simulink model "Gesamtsystem_VirtuelleTestUmgebung"  (R2018b)
settings: Solver=FixedStepDiscrete  StartTime=0.0  StopTime=120  RelTol=1e-3  EnableMultiTasking=on
undefined symbols (not defined in the file): sigbuilder_block
libraries: simulink x2
settings Model: ExtModeTrigDuration=8  Creator=Nici  LastModifiedBy=Nici
settings SolverCC: AutoInsertRateTranBlk=on
settings OptimizationCC: DefaultUnderspecifiedDataType=single  EnhancedBackFolding=on  PassReuseOutputArgsAs=Individual arguments  MaxStackSize=512  OptimizeBlockOrder=speed  DifferentSizesBufferReuse=on  OptimizationCustomize=off
settings DebuggingCC: ParameterTunabilityLossMsg=error  UnderSpecifiedDataTypeMsg=warning
settings HardwareCC: ProdBitPerChar=16  ProdBitPerInt=16  ProdBitPerPointer=32  ProdBitPerSizeT=32  ProdBitPerPtrDiffT=32  ProdLargestAtomicInteger=Integer  ProdLargestAtomicFloat=None  ProdWordSize=16  ProdLongLongMode=on  ProdHWDeviceType=Texas Instruments->C2000
settings SFSimCC: MATLABDynamicMemAlloc=off
settings RTWCC: SystemTargetFile=ert.tlc  HardwareBoard=TI Delfino F2833x  TemplateMakefile=ert_default_tmf  GenerateReport=on  Toolchain=Texas Instruments Code Composer Studio (C2000)  IncludeHyperlinkInReport=on  LaunchReport=on  GenerateTraceInfo=on  GenerateTraceReport=on  GenerateTraceReportSl=on  GenerateTraceReportSf=on  GenerateTraceReportEml=on
settings CodeAppCC: ForceParamTrailComments=on  IgnoreCustomStorageClasses=off  OperatorAnnotations=on  SimulinkDataObjDesc=on  SFDataObjDesc=on  InsertBlockDesc=on
settings ERTTargetCC: CodeReplacementLibrary=TI C28x  SupportContinuousTime=on

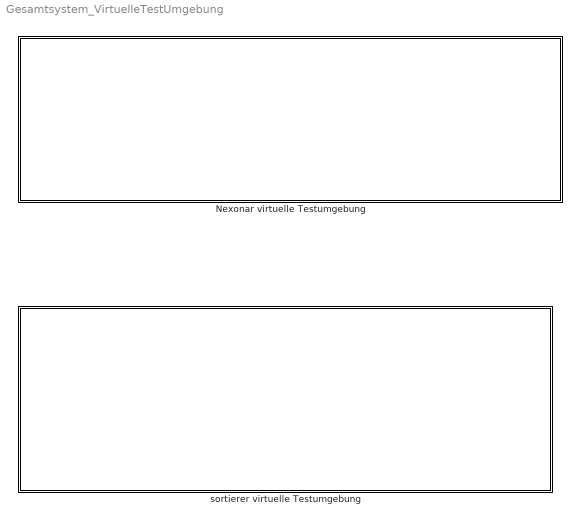
== system Gesamtsystem_VirtuelleTestUmgebung ==
  Nexonar virtuelle Testumgebung : Subsystem
  sortierer virtuelle Testumgebung : Subsystem

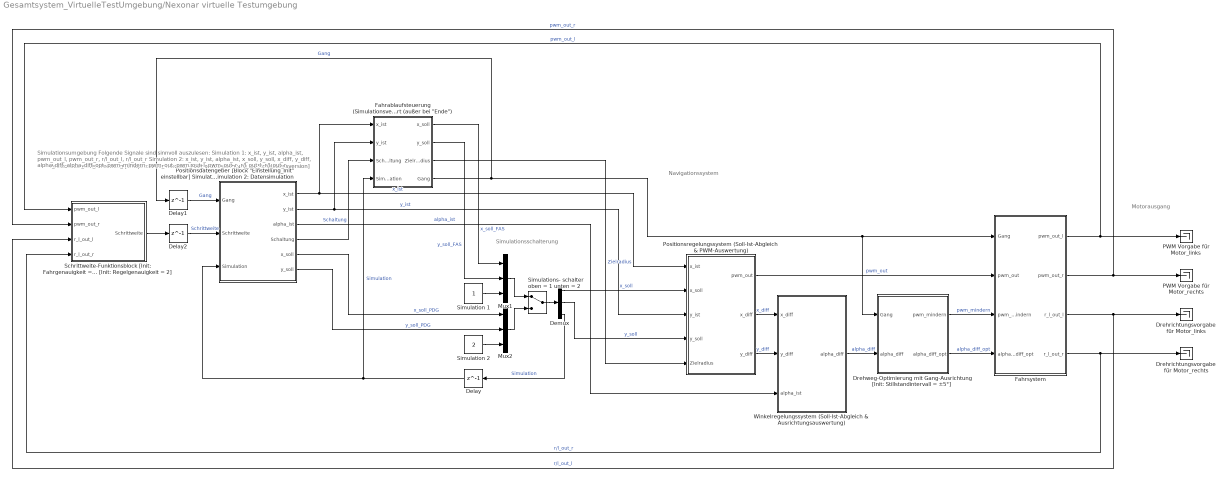
== system Gesamtsystem_VirtuelleTestUmgebung/Nexonar virtuelle Testumgebung ==
  note: Motorausgang
  note: Positionsdatenverarbeitung
      |
      |
      |
      |
      |
      |
      |
      |
      |
      |
      |
      |
      |
      |
      | [entspricht der Nexonar-Positionsbestimmung
      | als Simulationsversion]
  note: Simulationsschalterung
  note: Simulationsumgebung
      |
      |
      |
      |
      |
      |
      |
      |
      |
      |
      |
      |
      |
      |
      |
      |
      |
      |
      |
      |
      |
      |
      |
      |
      |
      |
      |
      |
      |
      |
      | Folgende Signale sind sinnvoll auszulesen:
      | Simulation 1: x_ist, y_ist, alpha_ist, pwm_out_l, pwm_out_r, r/l_out_l, r/l_out_r
      | Simulation 2: x_ist, y_ist, alpha_ist, x_soll, y_soll, x_diff, y_diff, alpha_diff, alpha_diff_opt, pwm_mindern, pwm_out, pwm_out_l, pwm_out_r, r/l_out_l, r/l_out_r
  note: Navigationssystem
  Delay : Delay  DelayLength=1  InitialCondition=0
  Delay1 : Delay  DelayLength=1  InitialCondition=0
  Delay2 : Delay  DelayLength=1  InitialCondition=0
  Demux : Demux  Outputs=3
  Drehrichtungsvorgabe für Motor_links : Terminator
  Drehrichtungsvorgabe für Motor_rechts : Terminator
  Drehweg-Optimierung mit Gang-Ausrichtung [Init: Stillstandintervall = ±5°] : Stateflow chart  TreatAsAtomicUnit=on
  "Fahrablaufsteuerung (Simulationsversion) [Init: Zielradius = 5mm] Gang = 0: vorwaerts Gang = 1: rueckwaerts Folgende Werte fuer den Ablauf sind einstellbar: - Zielkoordinatenwerte - Gangwert (außer bei \"Ende\")" : Stateflow chart  TreatAsAtomicUnit=on
  Fahrsystem : Stateflow chart  TreatAsAtomicUnit=on
  Mux1 : Mux  Inputs=3
  Mux2 : Mux  Inputs=3
  PWM Vorgabe für Motor_links : Terminator
  PWM Vorgabe für Motor_rechts : Terminator
  "Positionsdatengeber [Block \"Einstellung_Init\" einstellbar] Simulation 1: Fahrsimulation Simulation 2: Datensimulation" : Stateflow chart  TreatAsAtomicUnit=on
  Positionsregelungssystem (Soll-Ist-Abgleich & PWM-Auswertung) : Subsystem
  Schrittweite-Funktionsblock [Init: Fahrgenauigkeit = 10] [Init: Drehgenauigkeit = 30] [Init: Regelgenauigkeit = 2] : MATLAB Function  TreatAsAtomicUnit=on
  Simulation 1 : Constant
  Simulation 2 : Constant  Value=2
  Simulations- schalter oben = 1 unten = 2 : ManualSwitch
  Winkelregelungssystem (Soll-Ist-Abgleich & Ausrichtungsauswertung) : Subsystem
  wires:
  "Positionsdatengeber [Block \"Einstellung_Init\" einstellbar] Simulation 1: Fahrsimulation Simulation 2: Datensimulation"/1(x_ist) -> "Fahrablaufsteuerung (Simulationsversion) [Init: Zielradius = 5mm] Gang = 0: vorwaerts Gang = 1: rueckwaerts Folgende Werte fuer den Ablauf sind einstellbar: - Zielkoordinatenwerte - Gangwert (außer bei \"Ende\")"/1(x_ist), Positionsregelungssystem (Soll-Ist-Abgleich & PWM-Auswertung)/1(x_ist)  "x_ist"
  "Positionsdatengeber [Block \"Einstellung_Init\" einstellbar] Simulation 1: Fahrsimulation Simulation 2: Datensimulation"/2(y_ist) -> "Fahrablaufsteuerung (Simulationsversion) [Init: Zielradius = 5mm] Gang = 0: vorwaerts Gang = 1: rueckwaerts Folgende Werte fuer den Ablauf sind einstellbar: - Zielkoordinatenwerte - Gangwert (außer bei \"Ende\")"/2(y_ist), Positionsregelungssystem (Soll-Ist-Abgleich & PWM-Auswertung)/3(y_ist)  "y_ist"
  "Fahrablaufsteuerung (Simulationsversion) [Init: Zielradius = 5mm] Gang = 0: vorwaerts Gang = 1: rueckwaerts Folgende Werte fuer den Ablauf sind einstellbar: - Zielkoordinatenwerte - Gangwert (außer bei \"Ende\")"/2(y_soll) -> Mux1/2  "y_soll_FAS"
  Simulation 1/1 -> Mux1/3
  Positionsregelungssystem (Soll-Ist-Abgleich & PWM-Auswertung)/1(pwm_out) -> Fahrsystem/2(pwm_out)  "pwm_out"
  "Positionsdatengeber [Block \"Einstellung_Init\" einstellbar] Simulation 1: Fahrsimulation Simulation 2: Datensimulation"/4(Schaltung) -> "Fahrablaufsteuerung (Simulationsversion) [Init: Zielradius = 5mm] Gang = 0: vorwaerts Gang = 1: rueckwaerts Folgende Werte fuer den Ablauf sind einstellbar: - Zielkoordinatenwerte - Gangwert (außer bei \"Ende\")"/3(Schaltung)  "Schaltung"
  Delay2/1 -> "Positionsdatengeber [Block \"Einstellung_Init\" einstellbar] Simulation 1: Fahrsimulation Simulation 2: Datensimulation"/2(Schrittweite)  "Schrittweite"
  Delay1/1 -> "Positionsdatengeber [Block \"Einstellung_Init\" einstellbar] Simulation 1: Fahrsimulation Simulation 2: Datensimulation"/1(Gang)  "Gang"
  "Positionsdatengeber [Block \"Einstellung_Init\" einstellbar] Simulation 1: Fahrsimulation Simulation 2: Datensimulation"/3(alpha_ist) -> Winkelregelungssystem (Soll-Ist-Abgleich & Ausrichtungsauswertung)/3(alpha_ist)  "alpha_ist"
  "Positionsdatengeber [Block \"Einstellung_Init\" einstellbar] Simulation 1: Fahrsimulation Simulation 2: Datensimulation"/5(x_soll) -> Mux2/1  "x_soll_PDG"
  Delay/1 -> "Positionsdatengeber [Block \"Einstellung_Init\" einstellbar] Simulation 1: Fahrsimulation Simulation 2: Datensimulation"/3(Simulation), "Fahrablaufsteuerung (Simulationsversion) [Init: Zielradius = 5mm] Gang = 0: vorwaerts Gang = 1: rueckwaerts Folgende Werte fuer den Ablauf sind einstellbar: - Zielkoordinatenwerte - Gangwert (außer bei \"Ende\")"/4(Simulation)  "Simulation"
  "Positionsdatengeber [Block \"Einstellung_Init\" einstellbar] Simulation 1: Fahrsimulation Simulation 2: Datensimulation"/6(y_soll) -> Mux2/2  "y_soll_PDG"
  Drehweg-Optimierung mit Gang-Ausrichtung [Init: Stillstandintervall = ±5°]/2(alpha_diff_opt) -> Fahrsystem/4(alpha_diff_opt)  "alpha_diff_opt"
  Winkelregelungssystem (Soll-Ist-Abgleich & Ausrichtungsauswertung)/1(alpha_diff) -> Drehweg-Optimierung mit Gang-Ausrichtung [Init: Stillstandintervall = ±5°]/2(alpha_diff)  "alpha_diff"
  Fahrsystem/4(r_l_out_r) -> Schrittweite-Funktionsblock [Init: Fahrgenauigkeit = 10] [Init: Drehgenauigkeit = 30] [Init: Regelgenauigkeit = 2]/4(r_l_out_r), Drehrichtungsvorgabe für Motor_rechts/1  "r/l_out_r"
  Mux1/1 -> Simulations- schalter oben = 1 unten = 2/1
  Demux/2 -> Positionsregelungssystem (Soll-Ist-Abgleich & PWM-Auswertung)/4(y_soll)  "y_soll"
  Positionsregelungssystem (Soll-Ist-Abgleich & PWM-Auswertung)/2(x_diff) -> Winkelregelungssystem (Soll-Ist-Abgleich & Ausrichtungsauswertung)/1(x_diff)  "x_diff"
  Fahrsystem/3(r_l_out_l) -> Drehrichtungsvorgabe für Motor_links/1, Schrittweite-Funktionsblock [Init: Fahrgenauigkeit = 10] [Init: Drehgenauigkeit = 30] [Init: Regelgenauigkeit = 2]/3(r_l_out_l)  "r/l_out_l"
  Simulations- schalter oben = 1 unten = 2/1 -> Demux/1
  "Fahrablaufsteuerung (Simulationsversion) [Init: Zielradius = 5mm] Gang = 0: vorwaerts Gang = 1: rueckwaerts Folgende Werte fuer den Ablauf sind einstellbar: - Zielkoordinatenwerte - Gangwert (außer bei \"Ende\")"/4(Gang) -> Drehweg-Optimierung mit Gang-Ausrichtung [Init: Stillstandintervall = ±5°]/1(Gang), Fahrsystem/1(Gang), Delay1/1  "Gang"
  "Fahrablaufsteuerung (Simulationsversion) [Init: Zielradius = 5mm] Gang = 0: vorwaerts Gang = 1: rueckwaerts Folgende Werte fuer den Ablauf sind einstellbar: - Zielkoordinatenwerte - Gangwert (außer bei \"Ende\")"/3(Zielradius) -> Positionsregelungssystem (Soll-Ist-Abgleich & PWM-Auswertung)/5(Zielradius)  "Zielradius"
  Fahrsystem/1(pwm_out_l) -> PWM Vorgabe für Motor_links/1, Schrittweite-Funktionsblock [Init: Fahrgenauigkeit = 10] [Init: Drehgenauigkeit = 30] [Init: Regelgenauigkeit = 2]/1(pwm_out_l)  "pwm_out_l"
  Simulation 2/1 -> Mux2/3
  "Fahrablaufsteuerung (Simulationsversion) [Init: Zielradius = 5mm] Gang = 0: vorwaerts Gang = 1: rueckwaerts Folgende Werte fuer den Ablauf sind einstellbar: - Zielkoordinatenwerte - Gangwert (außer bei \"Ende\")"/1(x_soll) -> Mux1/1  "x_soll_FAS"
  Schrittweite-Funktionsblock [Init: Fahrgenauigkeit = 10] [Init: Drehgenauigkeit = 30] [Init: Regelgenauigkeit = 2]/1(Schrittweite) -> Delay2/1
  Positionsregelungssystem (Soll-Ist-Abgleich & PWM-Auswertung)/3(y_diff) -> Winkelregelungssystem (Soll-Ist-Abgleich & Ausrichtungsauswertung)/2(y_diff)  "y_diff"
  Demux/1 -> Positionsregelungssystem (Soll-Ist-Abgleich & PWM-Auswertung)/2(x_soll)  "x_soll"
  Demux/3 -> Delay/1  "Simulation"
  Drehweg-Optimierung mit Gang-Ausrichtung [Init: Stillstandintervall = ±5°]/1(pwm_mindern) -> Fahrsystem/3(pwm_mindern)  "pwm_mindern"
  Fahrsystem/2(pwm_out_r) -> PWM Vorgabe für Motor_rechts/1, Schrittweite-Funktionsblock [Init: Fahrgenauigkeit = 10] [Init: Drehgenauigkeit = 30] [Init: Regelgenauigkeit = 2]/2(pwm_out_r)  "pwm_out_r"
  Mux2/1 -> Simulations- schalter oben = 1 unten = 2/2

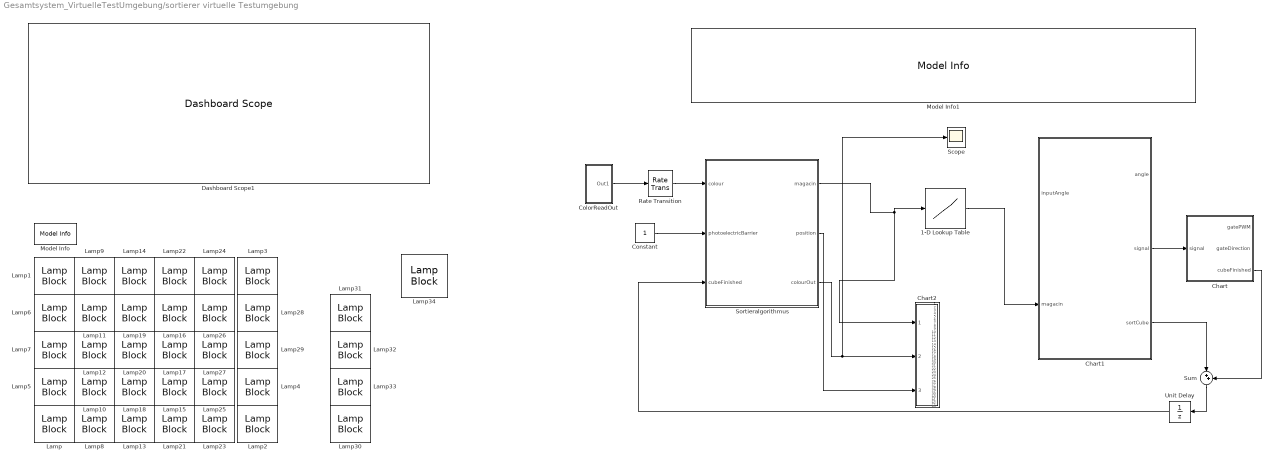
== system Gesamtsystem_VirtuelleTestUmgebung/sortierer virtuelle Testumgebung ==
  1-D Lookup Table : Lookup_n-D  NumberOfTableDimensions=1  BreakpointsForDimension1=[-1,0,1,2,3,4,5,6]  Table=[-1,-440,-295,-170,-40,85,220,430]  InternalRulePriority=Speed  RndMeth=Simplest  InputSameDT=on
  Chart : Stateflow chart  TreatAsAtomicUnit=on
  Chart1 : Stateflow chart  TreatAsAtomicUnit=on
  Chart2 : Stateflow chart  TreatAsAtomicUnit=on
  ColorReadOut : Subsystem
  Constant : Constant
  Dashboard Scope1 : DashboardScope  WebBlockId=334  Ymin=-450  Ymax=450
  Lamp : LampBlock  WebBlockId=336  LabelPosition=Hide
  Lamp1 : LampBlock  WebBlockId=337  LabelPosition=Hide
  Lamp10 : LampBlock  WebBlockId=338  LabelPosition=Hide
  Lamp11 : LampBlock  WebBlockId=339  LabelPosition=Hide
  Lamp12 : LampBlock  WebBlockId=340  LabelPosition=Hide
  Lamp13 : LampBlock  WebBlockId=341  LabelPosition=Hide
  Lamp14 : LampBlock  WebBlockId=342  LabelPosition=Hide
  Lamp15 : LampBlock  WebBlockId=343  LabelPosition=Hide
  Lamp16 : LampBlock  WebBlockId=344  LabelPosition=Hide
  Lamp17 : LampBlock  WebBlockId=345  LabelPosition=Hide
  Lamp18 : LampBlock  WebBlockId=346  LabelPosition=Hide
  Lamp19 : LampBlock  WebBlockId=347  LabelPosition=Hide
  Lamp2 : LampBlock  WebBlockId=348  LabelPosition=Hide
  Lamp20 : LampBlock  WebBlockId=349  LabelPosition=Hide
  Lamp21 : LampBlock  WebBlockId=350  LabelPosition=Hide
  Lamp22 : LampBlock  WebBlockId=351  LabelPosition=Hide
  Lamp23 : LampBlock  WebBlockId=352  LabelPosition=Hide
  Lamp24 : LampBlock  WebBlockId=353  LabelPosition=Hide
  Lamp25 : LampBlock  WebBlockId=354  LabelPosition=Hide
  Lamp26 : LampBlock  WebBlockId=355  LabelPosition=Hide
  Lamp27 : LampBlock  WebBlockId=356  LabelPosition=Hide
  Lamp28 : LampBlock  WebBlockId=357  LabelPosition=Hide
  Lamp29 : LampBlock  WebBlockId=358  LabelPosition=Hide
  Lamp3 : LampBlock  WebBlockId=359  LabelPosition=Hide
  Lamp30 : LampBlock  WebBlockId=360  LabelPosition=Hide
  Lamp31 : LampBlock  WebBlockId=361  LabelPosition=Hide
  Lamp32 : LampBlock  WebBlockId=362  LabelPosition=Hide
  Lamp33 : LampBlock  WebBlockId=363  LabelPosition=Hide
  Lamp34 : LampBlock  WebBlockId=364
  Lamp4 : LampBlock  WebBlockId=365  LabelPosition=Hide
  Lamp5 : LampBlock  WebBlockId=366  LabelPosition=Hide
  Lamp6 : LampBlock  WebBlockId=367  LabelPosition=Hide
  Lamp7 : LampBlock  WebBlockId=368  LabelPosition=Hide
  Lamp8 : LampBlock  WebBlockId=369  LabelPosition=Hide
  Lamp9 : LampBlock  WebBlockId=370  LabelPosition=Hide
  Model Info : simulink/Model-Wide Utilities/Model Info  Frame=on  DisplayStringWithTags=Magazin  HorizontalTextAlignment=Center  LeftAlignmentValue=0.5
  Model Info1 : simulink/Model-Wide Utilities/Model Info  Frame=on  DisplayStringWithTags=|  HorizontalTextAlignment=Center  LeftAlignmentValue=0.5
      | ReadMe
      | 
      | Um diese Testumgebung zum Laufen zu bringen, muss das Matlab Add On Real Time Pacer heruntergeladen und installiert werden. Der angefahrene InputAngle wurde hier als Delay
      | simuliert: sprich, es wird immer ein fester Zeitintervall angenommen, den der Motor braucht, um den Winkel anzufahren. 
      | 
      | Alle anderen Informationen zum genauen Ablauf des Algorithmus finden Sie auf der Dokumentation der Programmierung
  Rate Transition : RateTransition  InitialCondition=1  OutPortSampleTime=0.01
  Scope : Scope
  Sortieralgorithmus : Stateflow chart  TreatAsAtomicUnit=on
  Sum : Sum  Inputs=|++
  Unit Delay : UnitDelay  SampleTime=-1
  wires:
  Sortieralgorithmus/2(position) -> Chart2/3(position)
  Chart/3(cubeFinished) -> Sum/2
  Chart1/3(sortCube) -> Sum/1
  Sortieralgorithmus/1(magacin) -> 1-D Lookup Table/1, Chart2/1(magacin)
  Chart1/2(signal) -> Chart/1(signal)
  Rate Transition/1 -> Sortieralgorithmus/1(colour)
  Constant/1 -> Sortieralgorithmus/2(photoelectricBarrier)
  Unit Delay/1 -> Sortieralgorithmus/3(cubeFinished)
  Sortieralgorithmus/3(colourOut) -> Scope/1, Chart2/2(colour)
  ColorReadOut/1(Out1) -> Rate Transition/1
  Sum/1 -> Unit Delay/1
  1-D Lookup Table/1 -> Chart1/2(magacin)

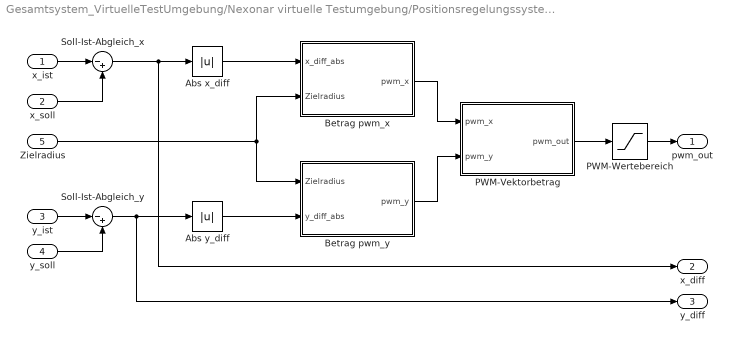
== system Gesamtsystem_VirtuelleTestUmgebung/Nexonar virtuelle Testumgebung/Positionsregelungssystem (Soll-Ist-Abgleich & PWM-Auswertung) ==
  x_ist : Inport
  x_soll : Inport  Port=2
  y_ist : Inport  Port=3
  y_soll : Inport  Port=4
  Zielradius : Inport  Port=5
  Abs x_diff : Abs  SampleTime=0.01
  Abs y_diff : Abs  SampleTime=0.01
  Betrag pwm_x : MATLAB Function  TreatAsAtomicUnit=on  SystemSampleTime=0.01
  Betrag pwm_y : MATLAB Function  TreatAsAtomicUnit=on  SystemSampleTime=0.01
  PWM-Vektorbetrag : MATLAB Function  TreatAsAtomicUnit=on
  PWM-Wertebereich : Saturate  UpperLimit=100  LowerLimit=0
  Soll-Ist-Abgleich_x : Sum  Inputs=|-+  SampleTime=0.01
  Soll-Ist-Abgleich_y : Sum  Inputs=|-+  AccumDataTypeStr=double  SampleTime=0.01
  pwm_out : Outport
  x_diff : Outport  Port=2
  y_diff : Outport  Port=3
  wires:
  Soll-Ist-Abgleich_x/1 -> x_diff/1, Abs x_diff/1
  Abs x_diff/1 -> Betrag pwm_x/1(x_diff_abs)
  x_soll/1 -> Soll-Ist-Abgleich_x/2
  x_ist/1 -> Soll-Ist-Abgleich_x/1
  y_ist/1 -> Soll-Ist-Abgleich_y/1
  y_soll/1 -> Soll-Ist-Abgleich_y/2
  Soll-Ist-Abgleich_y/1 -> Abs y_diff/1, y_diff/1
  Abs y_diff/1 -> Betrag pwm_y/2(y_diff_abs)
  PWM-Wertebereich/1 -> pwm_out/1
  PWM-Vektorbetrag/1(pwm_out) -> PWM-Wertebereich/1
  Betrag pwm_x/1(pwm_x) -> PWM-Vektorbetrag/1(pwm_x)
  Betrag pwm_y/1(pwm_y) -> PWM-Vektorbetrag/2(pwm_y)
  Zielradius/1 -> Betrag pwm_y/1(Zielradius), Betrag pwm_x/2(Zielradius)

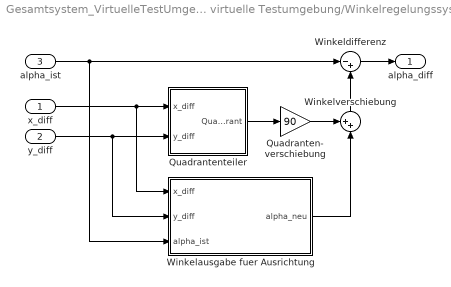
== system Gesamtsystem_VirtuelleTestUmgebung/Nexonar virtuelle Testumgebung/Winkelregelungssystem (Soll-Ist-Abgleich & Ausrichtungsauswertung) ==
  x_diff : Inport
  y_diff : Inport  Port=2
  alpha_ist : Inport  Port=3
  Quadranten- verschiebung : Gain  Gain=90
  Quadrantenteiler : Stateflow chart  TreatAsAtomicUnit=on
  Winkelausgabe fuer Ausrichtung : Stateflow chart  TreatAsAtomicUnit=on
  Winkeldifferenz : Sum  Inputs=|-+
  Winkelverschiebung : Sum  Inputs=++|
  alpha_diff : Outport
  wires:
  alpha_ist/1 -> Winkelausgabe fuer Ausrichtung/3(alpha_ist), Winkeldifferenz/1
  y_diff/1 -> Winkelausgabe fuer Ausrichtung/2(y_diff), Quadrantenteiler/2(y_diff)
  Winkelausgabe fuer Ausrichtung/1(alpha_neu) -> Winkelverschiebung/2
  Winkelverschiebung/1 -> Winkeldifferenz/2
  x_diff/1 -> Winkelausgabe fuer Ausrichtung/1(x_diff), Quadrantenteiler/1(x_diff)
  Quadrantenteiler/1(Quadrant) -> Quadranten- verschiebung/1
  Winkeldifferenz/1 -> alpha_diff/1
  Quadranten- verschiebung/1 -> Winkelverschiebung/1

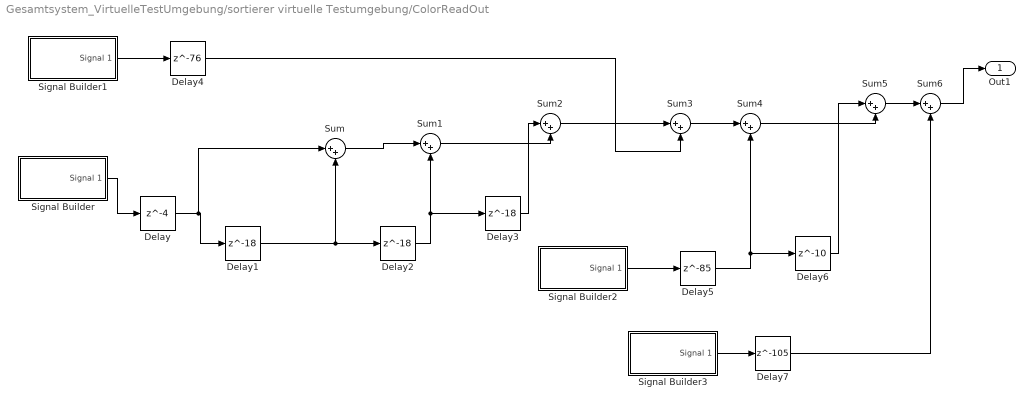
== system Gesamtsystem_VirtuelleTestUmgebung/sortierer virtuelle Testumgebung/ColorReadOut ==
  Delay : Delay  DelayLength=4  SampleTime=1
  Delay1 : Delay  DelayLength=18  SampleTime=1
  Delay2 : Delay  DelayLength=18  SampleTime=1
  Delay3 : Delay  DelayLength=18  SampleTime=1
  Delay4 : Delay  DelayLength=76  SampleTime=1
  Delay5 : Delay  DelayLength=85  SampleTime=1
  Delay6 : Delay  DelayLength=10  SampleTime=1
  Delay7 : Delay  DelayLength=105  SampleTime=1
  Signal Builder : Subsystem  Tag=STV Subsys  LoadFcn=sigbuilder_block('load');  StartFcn=sigbuilder_block('start');  StopFcn=sigbuilder_block('stop');  ClipboardFcn=sigbuilder_block('clipboard');  mask(Sigbuilder block){tuvar=[0:10]}
      mask help: Simulink:masks:SigbuilderBlock_MD
      mask init:
      | if ~strcmp(get_param(bdroot(gcbh),'SimulationStatus'),'stopped') tuvar = sigbuilder_block('maskInit'); end
      settings: CopyFcn=sigbuilder_block('copy');  DeleteFcn=sigbuilder_block('delete');  ModelCloseFcn=sigbuilder_block('modelClose');  PreSaveFcn=sigbuilder_block('preSave');  PauseFcn=sigbuilder_block('pause');  ContinueFcn=sigbuilder_block('continue');  NameChangeFcn=sigbuilder_block('namechange');  OpenFcn=sigbuilder_block('open',[404.625 154.25 550.5 330.5 ]);  CloseFcn=sigbuilder_block('close');
      mask Display: plot(0, 0, 100, 100,[2, 2, 32, 32, 2], [68, 8, 8, 68, 68],[32, 2], [38, 38], [32, 19, 2],[53, 60, 44], [32, 17, 17, 2],[16, 16, 31, 31]);txt = getActiveGroup(gcbh);text(2, 100, txt,'verticalAlignment', 'top');
  Signal Builder1 : Subsystem  Tag=STV Subsys  LoadFcn=sigbuilder_block('load');  StartFcn=sigbuilder_block('start');  StopFcn=sigbuilder_block('stop');  ClipboardFcn=sigbuilder_block('clipboard');  mask(Sigbuilder block){tuvar=[0:10]}
      mask help: Simulink:masks:SigbuilderBlock_MD
      mask init:
      | if ~strcmp(get_param(bdroot(gcbh),'SimulationStatus'),'stopped') tuvar = sigbuilder_block('maskInit'); end
      settings: CopyFcn=sigbuilder_block('copy');  DeleteFcn=sigbuilder_block('delete');  ModelCloseFcn=sigbuilder_block('modelClose');  PreSaveFcn=sigbuilder_block('preSave');  PauseFcn=sigbuilder_block('pause');  ContinueFcn=sigbuilder_block('continue');  NameChangeFcn=sigbuilder_block('namechange');  OpenFcn=sigbuilder_block('open',[404.625 154.25 550.5 330.5 ]);  CloseFcn=sigbuilder_block('close');
      mask Display: plot(0, 0, 100, 100,[2, 2, 32, 32, 2], [68, 8, 8, 68, 68],[32, 2], [38, 38], [32, 19, 2],[53, 60, 44], [32, 17, 17, 2],[16, 16, 31, 31]);txt = getActiveGroup(gcbh);text(2, 100, txt,'verticalAlignment', 'top');
  Signal Builder2 : Subsystem  Tag=STV Subsys  LoadFcn=sigbuilder_block('load');  StartFcn=sigbuilder_block('start');  StopFcn=sigbuilder_block('stop');  ClipboardFcn=sigbuilder_block('clipboard');  mask(Sigbuilder block){tuvar=[0:10]}
      mask help: Simulink:masks:SigbuilderBlock_MD
      mask init:
      | if ~strcmp(get_param(bdroot(gcbh),'SimulationStatus'),'stopped') tuvar = sigbuilder_block('maskInit'); end
      settings: CopyFcn=sigbuilder_block('copy');  DeleteFcn=sigbuilder_block('delete');  ModelCloseFcn=sigbuilder_block('modelClose');  PreSaveFcn=sigbuilder_block('preSave');  PauseFcn=sigbuilder_block('pause');  ContinueFcn=sigbuilder_block('continue');  NameChangeFcn=sigbuilder_block('namechange');  OpenFcn=sigbuilder_block('open',[190.875 143.25 550.5 330.75 ]);  CloseFcn=sigbuilder_block('close');
      mask Display: plot(0, 0, 100, 100,[2, 2, 32, 32, 2], [68, 8, 8, 68, 68],[32, 2], [38, 38], [32, 19, 2],[53, 60, 44], [32, 17, 17, 2],[16, 16, 31, 31]);txt = getActiveGroup(gcbh);text(2, 100, txt,'verticalAlignment', 'top');
  Signal Builder3 : Subsystem  Tag=STV Subsys  LoadFcn=sigbuilder_block('load');  StartFcn=sigbuilder_block('start');  StopFcn=sigbuilder_block('stop');  ClipboardFcn=sigbuilder_block('clipboard');  mask(Sigbuilder block){tuvar=[0:10]}
      mask help: Simulink:masks:SigbuilderBlock_MD
      mask init:
      | if ~strcmp(get_param(bdroot(gcbh),'SimulationStatus'),'stopped') tuvar = sigbuilder_block('maskInit'); end
      settings: CopyFcn=sigbuilder_block('copy');  DeleteFcn=sigbuilder_block('delete');  ModelCloseFcn=sigbuilder_block('modelClose');  PreSaveFcn=sigbuilder_block('preSave');  PauseFcn=sigbuilder_block('pause');  ContinueFcn=sigbuilder_block('continue');  NameChangeFcn=sigbuilder_block('namechange');  OpenFcn=sigbuilder_block('open',[190.875 143.25 550.5 330.75 ]);  CloseFcn=sigbuilder_block('close');
      mask Display: plot(0, 0, 100, 100,[2, 2, 32, 32, 2], [68, 8, 8, 68, 68],[32, 2], [38, 38], [32, 19, 2],[53, 60, 44], [32, 17, 17, 2],[16, 16, 31, 31]);txt = getActiveGroup(gcbh);text(2, 100, txt,'verticalAlignment', 'top');
  Sum{,1..6} (7 alike) : Sum  Inputs=|++
  Out1 : Outport
  wires:
  Delay3/1 -> Sum2/1
  Sum/1 -> Sum1/1
  Signal Builder/1(Signal 1) -> Delay/1
  Sum1/1 -> Sum2/2
  Delay2/1 -> Delay3/1, Sum1/2
  Delay1/1 -> Delay2/1, Sum/2
  Delay/1 -> Sum/1, Delay1/1
  Sum2/1 -> Sum3/1
  Signal Builder1/1(Signal 1) -> Delay4/1
  Delay4/1 -> Sum3/2
  Signal Builder2/1(Signal 1) -> Delay5/1
  Delay5/1 -> Delay6/1, Sum4/2
  Sum3/1 -> Sum4/1
  Delay6/1 -> Sum5/1
  Sum4/1 -> Sum5/2
  Signal Builder3/1(Signal 1) -> Delay7/1
  Sum6/1 -> Out1/1
  Sum5/1 -> Sum6/1
  Delay7/1 -> Sum6/2

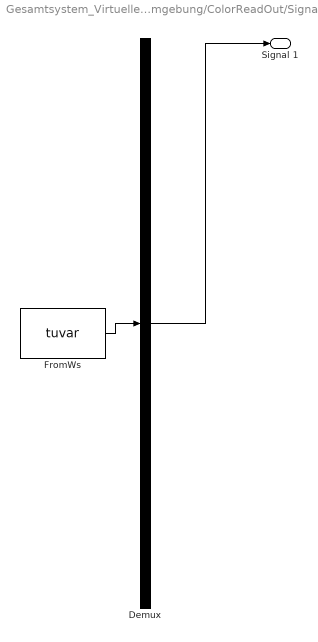
== system Gesamtsystem_VirtuelleTestUmgebung/sortierer virtuelle Testumgebung/ColorReadOut/Signal Builder ==
  Demux : Demux  Tag=STV Demux  Outputs=1
  FromWs : FromWorkspace  Tag=STV FromWs  VariableName=tuvar  SampleTime=0
      SigBuilderData=|
      | common.afterFinalStr = 'Extrapolate'
      | common.sampleTime = 0
      | dataSet.timeRange = [0 30]
      | dataSet.name = 'Group 1'
      | sbobj.Groups.Name = 'Group 1'
      | sbobj.Groups.Signals.Name = 'Signal 1'
      | sbobj.Groups.Signals.XData = [0 1 1 3 3 4 4 6 6 7 7 9 9 10 10 12 12 13 13 15 15 16 16 21.5 23.3 24.55 25.55 26.7 28.05 30]
      | sbobj.Groups.Signals.YData = [1800 1800 0 0 1800 1800 0 0 2700 2700 0 0 200 200 0 0 1800 1800 0 0 250 250 0 0 0 0 0 0 0 0]
      | sbobj.Groups.TimeRange = [0 30]
  Signal 1 : Outport  Tag=STV Outport
  wires:
  Demux/1 -> Signal 1/1
  FromWs/1 -> Demux/1

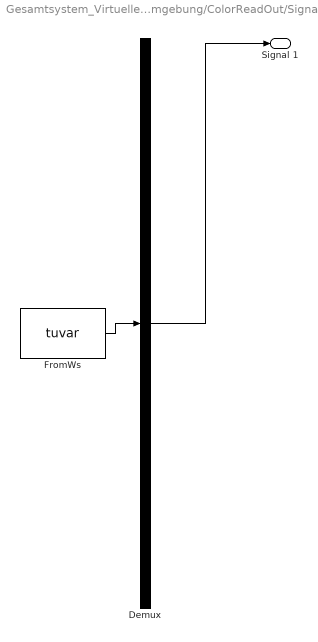
== system Gesamtsystem_VirtuelleTestUmgebung/sortierer virtuelle Testumgebung/ColorReadOut/Signal Builder1 ==
  Demux : Demux  Tag=STV Demux  Outputs=1
  FromWs : FromWorkspace  Tag=STV FromWs  VariableName=tuvar  SampleTime=0
      SigBuilderData=|
      | common.afterFinalStr = 'Extrapolate'
      | common.sampleTime = 0
      | dataSet.timeRange = [0 30]
      | dataSet.name = 'Group 1'
      | sbobj.Groups.Name = 'Group 1'
      | sbobj.Groups.Signals.Name = 'Signal 1'
      | sbobj.Groups.Signals.XData = [0 1 1 3 3 4 4 6 6 7 7 9 12 21.5 23.3 24.55 25.55 26.7 28.05 30]
      | sbobj.Groups.Signals.YData = [1800 1800 0 0 1800 1800 0 0 250 250 0 0 0 0 0 0 0 0 0 0]
      | sbobj.Groups.TimeRange = [0 30]
  Signal 1 : Outport  Tag=STV Outport
  wires:
  Demux/1 -> Signal 1/1
  FromWs/1 -> Demux/1

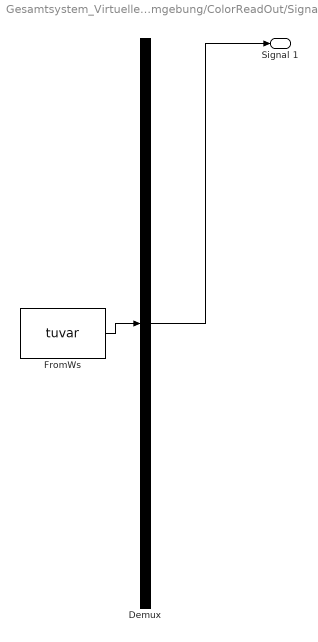
== system Gesamtsystem_VirtuelleTestUmgebung/sortierer virtuelle Testumgebung/ColorReadOut/Signal Builder2 ==
  Demux : Demux  Tag=STV Demux  Outputs=1
  FromWs : FromWorkspace  Tag=STV FromWs  VariableName=tuvar  SampleTime=0
      SigBuilderData=|
      | common.afterFinalStr = 'Extrapolate'
      | common.sampleTime = 0
      | dataSet.timeRange = [0 30]
      | dataSet.name = 'Group 1'
      | sbobj.Groups.Name = 'Group 1'
      | sbobj.Groups.Signals.Name = 'Signal 1'
      | sbobj.Groups.Signals.XData = [0 1 1 3 3 4 4 6 6 7 7 9 12 21.5 23.3 24.55 25.55 26.7 28.05 30]
      | sbobj.Groups.Signals.YData = [1800 1800 0 0 1800 1800 0 0 1800 1800 0 0 0 0 0 0 0 0 0 0]
      | sbobj.Groups.TimeRange = [0 30]
  Signal 1 : Outport  Tag=STV Outport
  wires:
  Demux/1 -> Signal 1/1
  FromWs/1 -> Demux/1

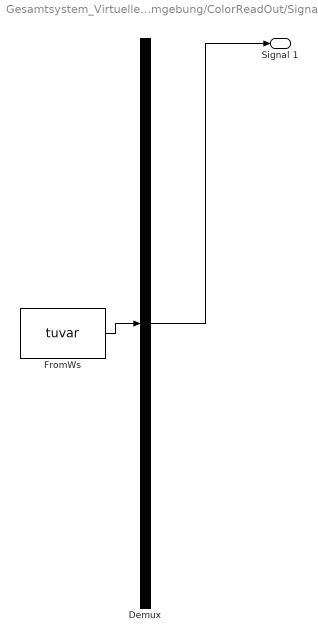
== system Gesamtsystem_VirtuelleTestUmgebung/sortierer virtuelle Testumgebung/ColorReadOut/Signal Builder3 ==
  Demux : Demux  Tag=STV Demux  Outputs=1
  FromWs : FromWorkspace  Tag=STV FromWs  VariableName=tuvar  SampleTime=0
      SigBuilderData=|
      | common.afterFinalStr = 'Extrapolate'
      | common.sampleTime = 0
      | dataSet.timeRange = [0 30]
      | dataSet.name = 'Group 1'
      | sbobj.Groups.Name = 'Group 1'
      | sbobj.Groups.Signals.Name = 'Signal 1'
      | sbobj.Groups.Signals.XData = [0 1 1 7 9 12 21.5 23.3 24.55 25.55 26.7 28.05 30]
      | sbobj.Groups.Signals.YData = [1800 1800 0 0 0 0 0 0 0 0 0 0 0]
      | sbobj.Groups.TimeRange = [0 30]
  Signal 1 : Outport  Tag=STV Outport
  wires:
  Demux/1 -> Signal 1/1
  FromWs/1 -> Demux/1

== stateflow chart Gesamtsystem_VirtuelleTestUmgebung/Nexonar virtuelle Testumgebung/Fahrablaufsteuerung (Simulationsversion) [Init: Zielradius = 5mm] Gang = 0: vorwaerts Gang = 1: rueckwaerts Folgende Werte fuer den Ablauf sind einstellbar: - Zielkoordinatenwerte - Gangwert (außer bei "Ende") ==
  state Start_Einstellung_Init
    entry:
    Zielradius = 5;
  state Parken
    entry:
    x_soll = x_least;
    y_soll = -100;
  state Uebergabe
    state Uebergabepunkt_x_Richtung
      entry:
      x_soll = x_least;
      y_soll = y_least;
    state Wechsel_1
      entry:
      Counter = Counter + 1;
    state Uebergabepunkt_y_Richtung
      entry:
      x_soll = x_least;
      y_soll = 100;
    state Wechsel_2
      entry:
      Counter = Counter + 1;
    (default) -> Uebergabepunkt_x_Richtung : {Counter = 0}
    Uebergabepunkt_x_Richtung -> Uebergabe.Wechsel_1 : [abs(x_soll - x_ist) <= Zielradius && abs(y_soll - y_ist) <= Zielradius]
        | {x_least = x_soll; y_least = y_soll;}
    Uebergabe.Wechsel_1 -> Uebergabepunkt_y_Richtung
    Uebergabepunkt_y_Richtung -> Uebergabe.Wechsel_2 : [abs(x_soll - x_ist) <= Zielradius && abs(y_soll - y_ist) <= Zielradius]
  state Sammeln
    state Anfahrpunkt_1
      entry:
      x_soll = 1400;
      y_soll = 50;
    state Wechsel_1
      entry:
      Counter = Counter + 1;
    state Anfahrpunkt_2
      entry:
      x_soll = 800;
      y_soll = -50;
    state Wechsel_2
      entry:
      Counter = Counter + 1;
    state Anfahrpunkt_3
      entry:
      x_soll = 800;
      y_soll = 400;
    state Wechsel_3
      entry:
      Counter = Counter + 1;
    state Anfahrpunkt_4
      entry:
      x_soll = 950;
      y_soll = 550;
    state Wechsel_4
      entry:
      Counter = Counter + 1;
    state Anfahrpunkt_5
      entry:
      x_soll = 950;
      y_soll = 850;
    state Wechsel_5
      entry:
      Counter = Counter + 1;
    state Anfahrpunkt_6
      entry:
      x_soll = 400;
      y_soll = 800;
      Anfahrpunkt_6 -> Anfahrpunkt_6 [order 1]
    state Wechsel_6
      entry:
      Counter = Counter + 1;
    state Anfahrpunkt_7
      entry:
      x_soll = 300;
      y_soll = 650;
    state Wechsel_7
      entry:
      Counter = Counter + 1;
    state Anfahrpunkt_8
      entry:
      x_soll = 300;
      y_soll = 150;
    state Wechsel_8
      entry:
      Counter = Counter + 1;
    state Anfahrpunkt_9
      entry:
      x_soll = 200;
      y_soll = -50;
    state Wechsel_9
      entry:
      Counter = Counter + 1;
    state Anfahrpunkt_10
      entry:
      x_soll = 1450;
      y_soll = 50;
    state Wechsel_10
      entry:
      Counter = Counter + 1;
    (default) -> Anfahrpunkt_1 : {Counter = 0}
    Anfahrpunkt_1 -> Sammeln.Wechsel_1 : [abs(x_soll - x_ist) <= Zielradius && abs(y_soll - y_ist) <= Zielradius]
    Sammeln.Wechsel_1 -> Anfahrpunkt_2
    Anfahrpunkt_2 -> Sammeln.Wechsel_2 : [abs(x_soll - x_ist) <= Zielradius && abs(y_soll - y_ist) <= Zielradius]
    Sammeln.Wechsel_2 -> Anfahrpunkt_3
    Anfahrpunkt_3 -> Wechsel_3 : [abs(x_soll - x_ist) <= Zielradius && abs(y_soll - y_ist) <= Zielradius]
    Wechsel_3 -> Anfahrpunkt_4
    Anfahrpunkt_4 -> Wechsel_4 : [abs(x_soll - x_ist) <= Zielradius && abs(y_soll - y_ist) <= Zielradius]
    Wechsel_4 -> Anfahrpunkt_5
    Anfahrpunkt_5 -> Wechsel_5 : [abs(x_soll - x_ist) <= Zielradius && abs(y_soll - y_ist) <= Zielradius]
    Wechsel_5 -> Anfahrpunkt_6
    Anfahrpunkt_6 -> Wechsel_6 [order 1] : [abs(x_soll - x_ist) <= Zielradius && abs(y_soll - y_ist) <= Zielradius]
    Wechsel_6 -> Anfahrpunkt_7
    Anfahrpunkt_7 -> Wechsel_7 : [abs(x_soll - x_ist) <= Zielradius && abs(y_soll - y_ist) <= Zielradius]
    Wechsel_7 -> Anfahrpunkt_8
    Anfahrpunkt_8 -> Wechsel_8 : [abs(x_soll - x_ist) <= Zielradius && abs(y_soll - y_ist) <= Zielradius]
    Wechsel_8 -> Anfahrpunkt_9
    Anfahrpunkt_9 -> Wechsel_9 : [abs(x_soll - x_ist) <= Zielradius && abs(y_soll - y_ist) <= Zielradius]
    Wechsel_9 -> Anfahrpunkt_10
    Anfahrpunkt_10 -> Wechsel_10 : [abs(x_soll - x_ist) <= Zielradius && abs(y_soll - y_ist) <= Zielradius]
  state Schaltung_Gang_Weiterleitung
    Gang = Schaltung;
  state Ende
    entry:
    Gang = 2;
  (default) -> Start_Einstellung_Init
  Start_Einstellung_Init -> (junction 137)
  Schaltung_Gang_Weiterleitung -> Schaltung_Gang_Weiterleitung
  Uebergabe -> Parken : [Counter == 2]{Gang = 0}
  (junction 137) -> Schaltung_Gang_Weiterleitung [order 2]
  (junction 137) -> Sammeln [order 1] : [Simulation == 1]{Gang = 0}
  Sammeln -> Uebergabe : [Counter == 10]
      | {Gang = 1;
      | x_least = x_soll;
      | y_least = y_soll;}
  Parken -> Ende : [abs(x_soll - x_ist) <= Zielradius && abs(y_soll - y_ist) <= Zielradius]
  data: x_soll output; y_soll output; Zielradius output; x_ist input; y_ist input; Counter local; x_least local; y_least local; Schaltung input; Simulation input; Gang output

== matlab function Gesamtsystem_VirtuelleTestUmgebung/Nexonar virtuelle Testumgebung/Positionsregelungssystem (Soll-Ist-Abgleich & PWM-Auswertung)/PWM-Vektorbetrag ==
  data: pwm_x input; pwm_out output; pwm_y input
function pwm_out = fcn(pwm_x, pwm_y)

pwm_out = round(sqrt(pwm_x * pwm_x + pwm_y * pwm_y));

== stateflow chart Gesamtsystem_VirtuelleTestUmgebung/Nexonar virtuelle Testumgebung/Positionsdatengeber [Block "Einstellung_Init" einstellbar] Simulation 1: Fahrsimulation Simulation 2: Datensimulation ==
  state Einstellung_Init
    Start_x = 0;
    Start_y = 0;
    Start_alpha = 0; % nur 0 – 359 in Fahrsimulation
    %%%
    Anfang_x = 0;
    Anfang_y = 0;
    Pos_max = 1000;
    Winkel_max = 360;
    Pos_Schritt = 200;   % > 0
    Winkel_Schritt = 20; % > 0
  state Start
    x_ist = Start_x;
    x_soll = Anfang_x;
    y_ist = Start_y;
    y_soll = Anfang_y;
    alpha_ist = Start_alpha;
  state Fahrsimulation
    state Fahren_mit_Ausrichtungsregelung
      alpha_ist = alpha_ist + Schrittweite(2);
      x_ist = x_ist + round(Schrittweite(1) * cos(alpha_ist*2*pi/360+pi*Schaltung));
      y_ist = y_ist + round(Schrittweite(1) * sin(alpha_ist*2*pi/360+pi*Schaltung));
    state Drehen
      alpha_ist = alpha_ist + Schrittweite(2);
    (junction 190) -> (junction 192) [order 1] : [alpha_ist + Schrittweite(2) >= 360]
        | {alpha_ist = alpha_ist - 360}
    Fahren_mit_Ausrichtungsregelung -> (junction 138)
    (junction 192) -> Fahren_mit_Ausrichtungsregelung [order 2]
    (junction 190) -> (junction 192) [order 2] : [alpha_ist + Schrittweite(2) < 0]
        | {alpha_ist = alpha_ist + 360}
    (junction 190) -> (junction 192) [order 3]
    (default) -> (junction 190)
    Drehen -> (junction 138)
    (junction 192) -> Drehen [order 1] : [Schrittweite(1) == 0]
    (junction 138) -> (junction 190) : {Schaltung = Gang}
  state Ende
  state Datensimulation
    state x_ist_Counter
      x_ist = x_ist + Pos_Schritt;
    state x_soll_Counter
      x_soll = x_soll + Pos_Schritt;
    state alpha_ist_Counter
      alpha_ist = alpha_ist + Winkel_Schritt;
    state y_ist_Counter
      y_ist = y_ist + Pos_Schritt;
    state y_soll_Counter
      y_soll = y_soll + Pos_Schritt;
    state Gangwechsel
      Schaltung = Schaltung + 1;
    (junction 195) -> Gangwechsel [order 2] : [y_ist + Pos_Schritt > Pos_max && x_soll + Pos_Schritt > Pos_max && y_soll + Pos_Schritt > Pos_max && alpha_ist + Winkel_Schritt >= Winkel_max]
        | {x_ist = Start_x; y_ist = Start_y; x_soll = Anfang_x; y_soll = Anfang_y, alpha_ist = Start_alpha;}
    (junction 195) -> alpha_ist_Counter [order 3] : [y_ist + Pos_Schritt > Pos_max && x_soll + Pos_Schritt > Pos_max && y_soll + Pos_Schritt > Pos_max]
        | {x_ist = Start_x; y_ist = Start_y; x_soll = Anfang_x; y_soll = Anfang_y;}
    (default) -> (junction 195)
    (junction 195) -> y_soll_Counter [order 4] : [y_ist + Pos_Schritt > Pos_max && x_soll + Pos_Schritt > Pos_max]
        | {x_ist = Start_x; y_ist = Start_y;
        | x_soll = Anfang_x;}
    Gangwechsel -> (junction 195)
    alpha_ist_Counter -> (junction 195)
    y_soll_Counter -> (junction 195)
    (junction 195) -> x_soll_Counter [order 5] : [y_ist + Pos_Schritt > Pos_max]
        | {x_ist = Start_x;
        | y_ist = Start_y;}
    x_soll_Counter -> (junction 195)
    (junction 195) -> y_ist_Counter [order 6] : {x_ist = Start_x}
    y_ist_Counter -> (junction 195)
    (junction 195) -> x_ist_Counter [order 1] : [x_ist + Pos_Schritt <= Pos_max]
    x_ist_Counter -> (junction 195)
  (default) -> Einstellung_Init
  Einstellung_Init -> Start
  Start -> (junction 102)
  Fahrsimulation -> Ende : [Schaltung == 2]
  (junction 102) -> Fahrsimulation [order 1] : [Simulation == 1]{Schaltung = Gang}
  (junction 102) -> Datensimulation [order 2] : {Schaltung = 0}
  Datensimulation -> Ende : [Schaltung == 2]
  data: Gang input double; x_ist output; y_ist output; alpha_ist output; Schaltung output; x_soll output; y_soll output; Pos_max local; Pos_Schritt local; Winkel_Schritt local; Schrittweite input double; Simulation input; Start_x local; Start_y local; Start_alpha local; Anfang_x local; Anfang_y local; Winkel_max local

== stateflow chart Gesamtsystem_VirtuelleTestUmgebung/sortierer virtuelle Testumgebung/Chart ==
  state wait
    gatePWM = 0
    gateDirection = 1
    cubeFinished = 1
  state close
    gateDirection = 0
  state open
    gatePWM = 50
    cubeFinished = 0
  (default) -> wait
  wait -> open : [signal == 1]
  open -> close : [after(0.3,sec)]
  close -> wait : [after(0.3, sec)]
  data: signal input; gatePWM output; gateDirection output; cubeFinished output

== matlab function Gesamtsystem_VirtuelleTestUmgebung/Nexonar virtuelle Testumgebung/Schrittweite-Funktionsblock [Init: Fahrgenauigkeit = 10] [Init: Drehgenauigkeit = 30] [Init: Regelgenauigkeit = 2] ==
  data: pwm_out_l input; Schrittweite output; pwm_out_r input; r_l_out_l input; r_l_out_r input
function Schrittweite = fcn(pwm_out_l, pwm_out_r, r_l_out_l, r_l_out_r)

Fahrgenauigkeit = 10; % bis 100
Drehgenauigkeit = 30; % bis 100
Regelgenauigkeit = 3; % bis 5


Schrittweite = [0 0];
if r_l_out_l == r_l_out_r
    Schrittweite(1) = round(sqrt(pwm_out_l * pwm_out_l + pwm_out_r * pwm_out_r) / Fahrgenauigkeit);
    % Fahren Wertebereich brutto: 0 - 100
    Schrittweite(2) = round((pwm_out_r - pwm_out_l) / Regelgenauigkeit) * (1 + (r_l_out_l - 1) * 2);
    % Fahrregelung Wertebereich brutto: 0 - 5
else
    Schrittweite(1) = 0;
    Schrittweite(2) = round(sqrt(pwm_out_l * pwm_out_l + pwm_out_r * pwm_out_r) / Drehgenauigkeit) * (r_l_out_r - r_l_out_l);
    % Drehen Wertebereich brutto: 0 - 100
end

== stateflow chart Gesamtsystem_VirtuelleTestUmgebung/sortierer virtuelle Testumgebung/Chart1 ==
  state firstEntry
    entry: angle = 300;
  note: StartWinkel, da Schieber nicht in Mitte stehen darf am Anfang. 5 Sekunden Zeit um das Bord einzuschalten
  state waitForCube
  state goToZero
    angle = 0;
    sortCube = 1;
  state closeGate
    signal = 0
  state wait
  state openGate
    signal = 1
    sortCube = 0
  state goToMagacin
    entry: angle = magacin;
  (default) -> firstEntry
  firstEntry -> waitForCube : [after(3,sec)]
  closeGate -> waitForCube
  waitForCube -> goToZero : [magacin~= -1]
  goToZero -> wait : [after(1,sec)]
  openGate -> closeGate : [after(0.5, sec)]
  wait -> goToMagacin : [after(0.4, sec)]
  goToMagacin -> openGate : [after(1,sec)]
  data: inputAngle input; magacin input; angle output; signal output; sortCube output single

== stateflow chart Gesamtsystem_VirtuelleTestUmgebung/Nexonar virtuelle Testumgebung/Fahrsystem ==
  state Fahren_mit_Ausrichtungsregelung
    entry:
    pwm_out_l = pwm_out - round(pwm_mindern(1) * (pwm_out / 100) ^ 1.9) * l_mindern;
    pwm_out_r = pwm_out - round(pwm_mindern(1) * (pwm_out / 100) ^ 1.9) * r_mindern;
    r_l_out_l = 1 - Gang;
    r_l_out_r = 1 - Gang;
  state Start_Warten
  state Drehen_links_max
    entry:
    pwm_out_l = 100;
    pwm_out_r = 100;
    r_l_out_l = 0;
    r_l_out_r = 1;
  state Drehen_rechts_max
    entry:
    pwm_out_l = 100;
    pwm_out_r = 100;
    r_l_out_l = 1;
    r_l_out_r = 0;
  state Drehen_links_gesteuert
    entry:
    pwm_out_l = 59 + abs(alpha_diff_opt);
    pwm_out_r = 59 + abs(alpha_diff_opt);
    r_l_out_l = 0;
    r_l_out_r = 1;
  state Drehen_rechts_gesteuert
    entry:
    pwm_out_l = 59 + abs(alpha_diff_opt);
    pwm_out_r = 59 + abs(alpha_diff_opt);
    r_l_out_l = 1;
    r_l_out_r = 0;
  (junction 81) -> Fahren_mit_Ausrichtungsregelung [order 1] : [pwm_mindern(2) == 1]
      | {l_mindern = 1 - Gang; r_mindern = 0 + Gang;}
  (junction 81) -> Fahren_mit_Ausrichtungsregelung [order 2] : [pwm_mindern(2) == 0]
      | {l_mindern = 0 + Gang; r_mindern = 1 - Gang;}
  (junction 1) -> (junction 81) [order 2]
  Fahren_mit_Ausrichtungsregelung -> (junction 32)
  (junction 81) -> Fahren_mit_Ausrichtungsregelung [order 3] : {l_mindern = 0; r_mindern = 0;}
  Start_Warten -> (junction 1)
  (junction 32) -> (junction 1)
  (default) -> Start_Warten
  Drehen_links_max -> (junction 32)
  Drehen_rechts_max -> (junction 32)
  Drehen_links_gesteuert -> (junction 32)
  (junction 1) -> (junction 18) [order 1] : [abs(alpha_diff_opt) > 0 && pwm_out > 0]
  Drehen_rechts_gesteuert -> (junction 32)
  (junction 18) -> (junction 44) [order 1] : [abs(alpha_diff_opt) > 40]
  (junction 44) -> Drehen_links_max [order 1] : [alpha_diff_opt > 0]
  (junction 18) -> (junction 52) [order 2]
  (junction 44) -> Drehen_rechts_max [order 2]
  (junction 52) -> Drehen_links_gesteuert [order 1] : [alpha_diff_opt > 0]
  (junction 52) -> Drehen_rechts_gesteuert [order 2]
  data: Gang input; pwm_out input; pwm_mindern input; alpha_diff_opt input; pwm_out_l output; pwm_out_r output; r_l_out_l output; r_l_out_r output; l_mindern local; r_mindern local

== stateflow chart Gesamtsystem_VirtuelleTestUmgebung/Nexonar virtuelle Testumgebung/Drehweg-Optimierung mit Gang-Ausrichtung [Init: Stillstandintervall = ±5°] ==
  state Einstellung_Init
    entry:
    Stillstandintervall = 5;
    %
    pwm_mindern = [0 0];
  state Drehstillstand_mit_Ausrichtungsregelung
    entry:
    alpha_diff_opt = 0;
    if abs(alpha_diff_intern) < 5
    pwm_mindern(1) = round(abs(alpha_diff_intern) / 2);
    elseif abs(alpha_diff_intern) < 15
    pwm_mindern(1) = 3 + floor((abs(alpha_diff_intern) - 5) / 5);
    else
    pwm_mindern(1) = 5;
    end;
    if alpha_diff_intern < 0
    pwm_mindern(2) = 0;
    elseif alpha_diff_intern > 0
    pwm_mindern(2) = 1;
    else
    pwm_mindern(2) = 2;
    end;
  state Weiterleitung_bei_Drehzustand
    entry:
    alpha_diff_opt = alpha_diff_intern;
  (default) -> Einstellung_Init
  (junction 95) -> (junction 32)
  Einstellung_Init -> (junction 32)
  (junction 32) -> (junction 6) : {alpha_diff_intern = alpha_diff + 180 * Gang}
  (junction 6) -> (junction 68) [order 2]
  (junction 68) -> Drehstillstand_mit_Ausrichtungsregelung [order 1] : [abs(alpha_diff_intern) <= Stillstandintervall]
  Drehstillstand_mit_Ausrichtungsregelung -> (junction 95)
  (junction 6) -> (junction 13) [order 1] : [abs(alpha_diff_intern) > 180]
  (junction 13) -> (junction 68) [order 1] : [alpha_diff_intern > 0]
      | {alpha_diff_intern = -360 + alpha_diff_intern}
  Weiterleitung_bei_Drehzustand -> (junction 95)
  (junction 13) -> (junction 68) [order 2] : {alpha_diff_intern = 360 + alpha_diff_intern}
  (junction 68) -> Weiterleitung_bei_Drehzustand [order 2]
  data: pwm_mindern output; Gang input; alpha_diff input; alpha_diff_opt output; alpha_diff_intern local; Stillstandintervall local

== stateflow chart Gesamtsystem_VirtuelleTestUmgebung/sortierer virtuelle Testumgebung/Chart2 ==
  state Entry
    m11 = 0;
    m12 = 0;
    m13 = 0;
    m14 = 0;
    m15 = 0;
    m21 = 0;
    m22 = 0;
    m23 = 0;
    m24 = 0;
    m25 = 0;
    m31 = 0;
    m32 = 0;
    m33 = 0;
    m34 = 0;
    m35 = 0;
    m41 = 0;
    m42 = 0;
    m43  = 0;
    m44 = 0;
    m45 = 0;
    m51 = 0;
    m52 = 0;
    m53 = 0;
    m54 = 0;
    m55 = 0;
    m61 = 0;
    m62 = 0;
    m63 = 0;
    m64 = 0;
    m65 = 0;
    b1 = 0;
    b2 = 0;
    b3 = 0;
    b0 = 0;
  state Update
    updateColor()
  Entry -> Update
  (default) -> Entry
  data: m11 output; m12 output; m13 output; m14 output; m15 output; magacin input; colour input; position input; m21 output; m22 output; m23 output; m24 output; m25 output; m31 output; m32 output; m33 output; m34 output; m35 output; m41 output; m42 output; m44 output; m45 output; m43 output; m51 output; m52 output; m53 output; m54 output; m55 output; m61 output; m62 output; m63 output; m64 output; m65 output; b0 output; b1 output; b2 output; b3 output
  function updateColor:
    | function updateColor
    | 
    | 
    | 
    | if(magacin == 0)
    |     if(position == 1)
    |         m11 = colour;
    |     elseif(position == 2)
    |         m12 = colour;
    |     elseif(position == 3)
    |         m13 = colour;
    |     elseif(position == 4)
    |         m14 = colour;
    |     elseif(position == 5)
    |         m15 = colour;
    |     end
    | end
    | if(magacin == 1)
    |     if(position == 1)
    |         m21 = colour;
    |     elseif(position == 2)
    |         m22 = colour;
    |     elseif(position == 3)
    |         m23 = colour;
    |     elseif(position == 4)
    |         m24 = colour;
    |     elseif(position == 5)
    |         m25 = colour;
    |     end
    | end
    | if(magacin == 2)
    |     if(position == 1)
    |         m31 = colour;
    |     elseif(position == 2)
    |         m32 = colour;
    |     elseif(position == 3)
    |         m33 = colour;
    |     elseif(position == 4)
    |         m34 = colour;
    |     elseif(position == 5)
    |         m35 = colour;
    |     end
    | 
    | end
    | 
    | if(magacin == 3)
    |     if(position == 1)
    |         m41 = colour;
    |     elseif(position == 2)
    |         m42 = colour;
    |     elseif(position == 3)
    |         m43 = colour;
    |     elseif(position == 4)
    |         m44 = colour;
    |     elseif(position == 5)
    |         m45 = colour;
    |     end
    | 
    | end
    | 
    | if(magacin == 4)
    |     if(position == 1)
    |         m51 = colour;
    |     elseif(position == 2)
    |         m52 = colour;
    |     elseif(position == 3)
    |         m53 = colour;
    |     elseif(position == 4)
    |         m54 = colour;
    |     elseif(position == 5)
    |         m55 = colour;
    |     end
    | 
    | end
    | 
    | if(magacin == 5)
    |     if(position == 1)
    |         m61 = colour;
    |     elseif(position == 2)
    |         m62 = colour;
    |     elseif(position == 3)
    |         m63 = colour;
    |     elseif(position == 4)
    |         m64 = colour;
    |     elseif(position == 5)
    |         m65 = colour;
    |     end
    | end
    | 
    | if(colour == 3)
    |     if(position == 0)
    |         b0 = 1;
    |     elseif(position == 1)
    |         b1 = 1;
    |     elseif(position == 2)
    |         b2 = 1;
    |     elseif(position == 3)
    |         b3 = 1;
    |     end
    | end

== stateflow chart Gesamtsystem_VirtuelleTestUmgebung/sortierer virtuelle Testumgebung/Sortieralgorithmus ==
  state setupVariable
    magacin0 = 0;
    magacin1 = 0;
    magacin2 = 0;
    magacin3 = 0;
    magacin4 = 0;
    magacin5 = 0;
    magacin6 = 0;
    magacin0_LastCube = 0;
    magacin1_LastCube = 0;
    magacin2_LastCube = 0;
    magacin3_LastCube = 0;
    magacin4_LastCube = 0;
    magacin5_LastCube = 0;
    magacin6_LastCube = 0;
    magacin = -1;
    blacks = 0;
  state cubeLoaded
    magacin = -1;
  state photoelectricBarrierActivated
  state BlueCube
    entry: magacin = findPlaceForBlue();
    colourOut = 1;
  state RedCube
    entry: magacin = findPlaceForRed();
    colourOut = 2
  state Black
    magacin = 6;
    colourOut = 3;
    position = blacks;
    blacks = blacks + 1;
  state DetectedCube
  setupVariable -> cubeLoaded : [after (3, sec)]
  (default) -> setupVariable
  DetectedCube -> cubeLoaded : [cubeFinished == 0]
  cubeLoaded -> photoelectricBarrierActivated : [photoelectricBarrier < 400]
  photoelectricBarrierActivated -> BlueCube [order 2] : [((colour >= 1000) && (colour <= 2150)) ]
  photoelectricBarrierActivated -> RedCube [order 1] : [(colour < 2500) && (colour > 0)]
  RedCube -> DetectedCube
  BlueCube -> DetectedCube
  Black -> DetectedCube
  data: magacinOut function_output; magacinOut function_output; colour input; magacin6 local; magacin0_LastCube local; magacin3_LastCube local; magacin2_LastCube local; magacin5_LastCube local; magacin1_LastCube local; magacin6_LastCube local; magacin4_LastCube local; magacin output; photoelectricBarrier input; magacin0 local; magacin1 local; magacin2 local; magacin3 local; magacin4 local; magacin5 local; cubeFinished input; position output; colourOut output; blacks local
  function magacinOut  = findPlaceForRed:
    | function magacinOut  = findPlaceForRed
    | if((magacin1 == 0) || ((magacin1_LastCube == 1)&& (magacin1 < 5)))
    |             magacinOut = 1;
    |             magacin1 = magacin1 + 1;
    |             magacin1_LastCube = 2;
    |             position = magacin1;
    | elseif (((magacin2_LastCube == 1) && (magacin2 < 5)))
    |             magacinOut = 2;
    |             magacin2 = magacin2 + 1; 
    |             magacin2_LastCube = 2;
    |             position = magacin2;
    | elseif ((magacin0 < 5) && (magacin0 > 0))
    |             magacinOut = 0;
    |             magacin0 = magacin0 + 1;
    |             magacin0_LastCube = 2;
    |             position = magacin0;
    | else 
    |            
    |             magacinOut = 2;
    |             if(magacin3 < 5)
    |                 magacinOut = 3;
    |                 magacin3 = magacin3 + 1;
    |                 magacin3_LastCube = 2;
    |                 position = magacin3;
    |                 
    |             elseif(magacin4 < 5)
    |                 magacinOut = 4;
    |                 magacin4 = magacin4 + 1;
    |                 magacin4_LastCube = 2;
    |                 position = magacin4;
    |             elseif(magacin5 < 5)
    |                 magacinOut = 5;
    |                 magacin5 = magacin5 + 1;
    |                 magacin5_LastCube = 2;
    |                 position = magacin5;
    |                 
    |             elseif(magacin2 < 5)
    |                 magacinOut = 2;
    |                 magacin2 = magacin2 + 1;
    |                 magacin2_LastCube = 2;
    |                 position = magacin2;
    |             elseif(magacin2 < 5)
    |                 magacinOut = 2;
    |                 magacin2 = magacin2 + 1;
    |                 magacin2_LastCube = 2;
    |                 position = magacin2;
    |             elseif(magacin1 < 5)
    |                 magacinOut = 1;
    |                 magacin1 = magacin1 + 1;
    |                 magacin1_LastCube = 2;
    |                 position = magacin1;
    |                          
    |             end
    | 
    | end
  function magacinOut  = findPlaceForBlue:
    | function magacinOut  = findPlaceForBlue
    | 
    | %1 ist Code for Blue, 2 is Code for Red, 3 is Code for Black, 0 is empty
    | if(magacin0 == 0)  
    |             magacinOut = 0;
    |             magacin0 = (magacin0 + 1);
    |             magacin0_LastCube = 1;
    |             position = magacin0;
    | elseif ((magacin2 == 0) || (magacin2_LastCube == 2 && magacin2 < 5))
    |             magacinOut = 2;
    |             magacin2 = magacin2 + 1; 
    |             magacin2_LastCube = 1;
    |             position = magacin2;
    | elseif ((magacin1_LastCube == 2) && (magacin1 < 5))
    |             magacinOut = 1;
    |             magacin1 = magacin1 + 1;
    |             magacin1_LastCube = 1;
    |             position = magacin1;
    | elseif (magacin3 < 5)
    |             magacinOut = 3;
    |             magacin3 = (magacin3 + 1);
    |             position = magacin3;
    | elseif (magacin4 < 5)
    |             magacinOut = 4;
    |             magacin4 = (magacin4 + 1);
    |             position = magacin4;
    | else 
    |             magacinOut = 5;
    |             magacin5 = magacin5 + 1;
    |             position = magacin5;
    | end

== stateflow chart Gesamtsystem_VirtuelleTestUmgebung/Nexonar virtuelle Testumgebung/Winkelregelungssystem (Soll-Ist-Abgleich & Ausrichtungsauswertung)/Quadrantenteiler ==
  state Quadrant_a
    entry:
    Quadrant = 0;
  state Quadrant_b
    entry:
    Quadrant = 1;
  state Start_Warten
  state Quadrant_c
    entry:
    Quadrant = 2;
  state Quadrant_d
    entry:
    Quadrant = 3;
  (junction 6) -> Quadrant_a [order 1] : [x_diff >= 0 && y_diff >= 0]
  Quadrant_a -> (junction 35)
  (junction 6) -> Quadrant_b [order 2] : [x_diff <= 0 && y_diff > 0]
  Quadrant_b -> (junction 35)
  Start_Warten -> (junction 6)
  (junction 35) -> (junction 6)
  (default) -> Start_Warten
  (junction 6) -> Quadrant_c [order 3] : [x_diff < 0 && y_diff <= 0]
  Quadrant_c -> (junction 35)
  (junction 6) -> Quadrant_d [order 4]
  Quadrant_d -> (junction 35)
  data: x_diff input; y_diff input; Quadrant output

== stateflow chart Gesamtsystem_VirtuelleTestUmgebung/Nexonar virtuelle Testumgebung/Winkelregelungssystem (Soll-Ist-Abgleich & Ausrichtungsauswertung)/Winkelausgabe fuer Ausrichtung ==
  state Ausrichtung_ohne_Aenderung
    entry:
    alpha_neu = alpha_ist;
  state Start_Warten
  state Trigonometrische_Auswertung_in_Grad_fuer_Quadrant_1_3
    entry:
    alpha_neu = round(atan(abs(x_diff)/abs(y_diff))*360/(2*pi));
  state Trigonometrische_Auswertung_in_Grad_fuer_Quadrant_0_2
    entry:
    alpha_neu = round(atan(abs(y_diff)/abs(x_diff))*360/(2*pi));
  (junction 4) -> Ausrichtung_ohne_Aenderung [order 1] : [x_diff == 0 && y_diff == 0]
  Ausrichtung_ohne_Aenderung -> (junction 65)
  Start_Warten -> (junction 4)
  (junction 65) -> (junction 4)
  (default) -> Start_Warten
  (junction 4) -> Trigonometrische_Auswertung_in_Grad_fuer_Quadrant_1_3 [order 4]
  (junction 4) -> Trigonometrische_Auswertung_in_Grad_fuer_Quadrant_0_2 [order 2] : [x_diff > 0 && y_diff >= 0]
  Trigonometrische_Auswertung_in_Grad_fuer_Quadrant_0_2 -> (junction 65)
  (junction 4) -> Trigonometrische_Auswertung_in_Grad_fuer_Quadrant_0_2 [order 3] : [x_diff < 0 && y_diff <= 0]
  Trigonometrische_Auswertung_in_Grad_fuer_Quadrant_1_3 -> (junction 65)
  data: x_diff input; y_diff input; alpha_neu output; alpha_ist input

== matlab function Gesamtsystem_VirtuelleTestUmgebung/Nexonar virtuelle Testumgebung/Positionsregelungssystem (Soll-Ist-Abgleich & PWM-Auswertung)/Betrag pwm_x ==
  settings: updateMethod=DISCRETE  sampleTime=0.01
  data: x_diff_abs input; pwm_x output; Zielradius input
function pwm_x = fcn( x_diff_abs, Zielradius)

if Zielradius < x_diff_abs && x_diff_abs < 60 + Zielradius
    pwm_x = 60;
elseif x_diff_abs <= Zielradius
    pwm_x = 0;
elseif x_diff_abs >= 100 + Zielradius
    pwm_x = 100;
else
    pwm_x = x_diff_abs;
end

== matlab function Gesamtsystem_VirtuelleTestUmgebung/Nexonar virtuelle Testumgebung/Positionsregelungssystem (Soll-Ist-Abgleich & PWM-Auswertung)/Betrag pwm_y ==
  settings: updateMethod=DISCRETE  sampleTime=0.01
  data: Zielradius input; y_diff_abs input; pwm_y output
function pwm_y = fcn(Zielradius, y_diff_abs)

if Zielradius < y_diff_abs && y_diff_abs < 60 + Zielradius
    pwm_y = 60;
elseif y_diff_abs <= Zielradius
    pwm_y = 0;
elseif y_diff_abs >= 100 + Zielradius
    pwm_y = 100;
else
    pwm_y = y_diff_abs;
end
